simulink model "quest1"  (R2015a)
settings: Solver=ode45  StartTime=0.0  StopTime=20  RelTol=1e-3
libraries: simulink x1
settings Model: Creator=smishra  LastModifiedBy=Subodh

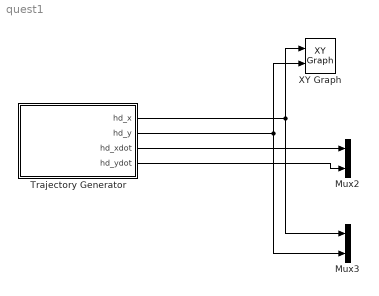
== system quest1 ==
  Mux2 : Mux  Inputs=2
  Mux3 : Mux  Inputs=2
  Trajectory Generator : Subsystem
  XY Graph : simulink/Sinks/XY Graph  xmin=0  xmax=3  ymin=0  ymax=3  st=-1
  wires:
  Trajectory Generator/1(hd_x) -> XY Graph/1, Mux3/1
  Trajectory Generator/2(hd_y) -> XY Graph/2, Mux3/2
  Trajectory Generator/3(hd_xdot) -> Mux2/1
  Trajectory Generator/4(hd_ydot) -> Mux2/2

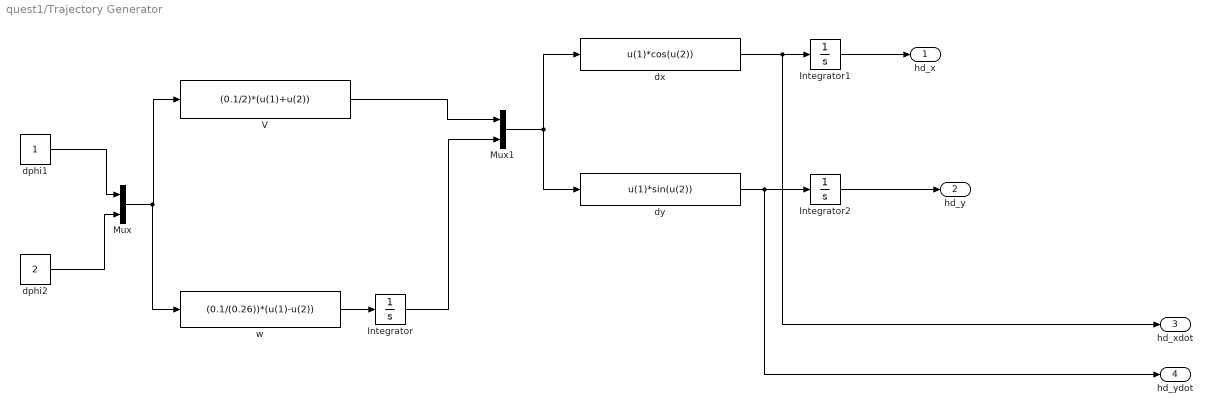
== system quest1/Trajectory Generator ==
  Integrator : Integrator  InitialCondition=3.141
  Integrator1 : Integrator  InitialCondition=2.3
  Integrator2 : Integrator
  Mux : Mux  Inputs=2
  Mux1 : Mux  Inputs=2
  V : Fcn  Expr=(0.1/2)*(u(1)+u(2))
  dphi1 : Constant
  dphi2 : Constant  Value=2
  dx : Fcn  Expr=u(1)*cos(u(2))
  dy : Fcn  Expr=u(1)*sin(u(2))
  w : Fcn  Expr=(0.1/(0.26))*(u(1)-u(2))
  hd_x : Outport
  hd_y : Outport  Port=2
  hd_xdot : Outport  Port=3
  hd_ydot : Outport  Port=4
  wires:
  Mux/1 -> w/1, V/1
  dphi2/1 -> Mux/2
  V/1 -> Mux1/1
  w/1 -> Integrator/1
  Mux1/1 -> dy/1, dx/1
  Integrator2/1 -> hd_y/1
  Integrator/1 -> Mux1/2
  dy/1 -> hd_ydot/1, Integrator2/1
  Integrator1/1 -> hd_x/1
  dphi1/1 -> Mux/1
  dx/1 -> hd_xdot/1, Integrator1/1
